simulink model "ModulationTutorial"  (R2017a)
settings: Solver=VariableStepAuto  StartTime=0.0  StopTime=10.0  RelTol=1e-3
libraries: dspsrcs4 x2
settings Model: Creator=cpelabws  LastModifiedBy=cpelabws

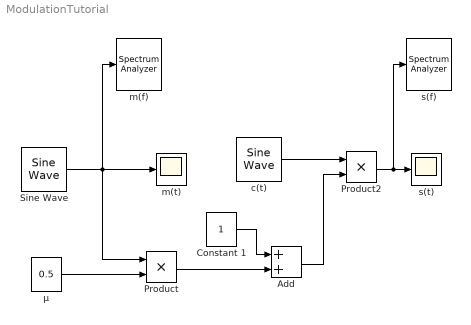
== system ModulationTutorial ==
  Add : Sum
  Constant 1 : Constant  VectorParams1D=off
  Product : Product
  Product2 : Product
  Sine Wave : dspsrcs4/Sine Wave  Amplitude=1  Frequency=5  Phase=0  SampleMode=Discrete  OutComplex=Real  CompMethod=Trigonometric fcn  TableSize=Speed  SampleTime=1/500  SamplesPerFrame=1  ResetState=Restart at time zero  OutputFrames=off  dataType=double  wordLen=16  udDataType=sfix(16)  fracBitsMode=Best precision  numFracBits=15  OutDataTypeStr=double  LastOutDataTypeStr=double
  "c(t) " : dspsrcs4/Sine Wave  Amplitude=1  Frequency=40  Phase=0  SampleMode=Discrete  OutComplex=Real  CompMethod=Trigonometric fcn  TableSize=Speed  SampleTime=1/500  SamplesPerFrame=1  ResetState=Restart at time zero  OutputFrames=off  dataType=double  wordLen=16  udDataType=sfix(16)  fracBitsMode=Best precision  numFracBits=15  OutDataTypeStr=double  LastOutDataTypeStr=double
  m(f) : SpectrumAnalyzer
  m(t) : Scope
  s(f) : SpectrumAnalyzer
  s(t) : Scope
  µ : Constant  Value=0.5  VectorParams1D=off
  wires:
  Sine Wave/1 -> m(f)/1, Product/1, m(t)/1
  µ/1 -> Product/2
  Product/1 -> Add/2
  Constant 1/1 -> Add/1
  "c(t) "/1 -> Product2/1
  Add/1 -> Product2/2
  Product2/1 -> s(f)/1, s(t)/1
